simulink model "Flight_Physics2_forTrim"  (R2017b)
settings: configuration reference "cs" (kept outside this file)
undefined symbols (not defined in the file or in its folder): Configuration, FOR_LDG_R_B, g, MOM_LDG_R_B, Ts
libraries: MathLibrary x2
settings Model: Creator=zht  LastModifiedBy=One
settings ConfigSetRef: SourceLocation=Base Workspace

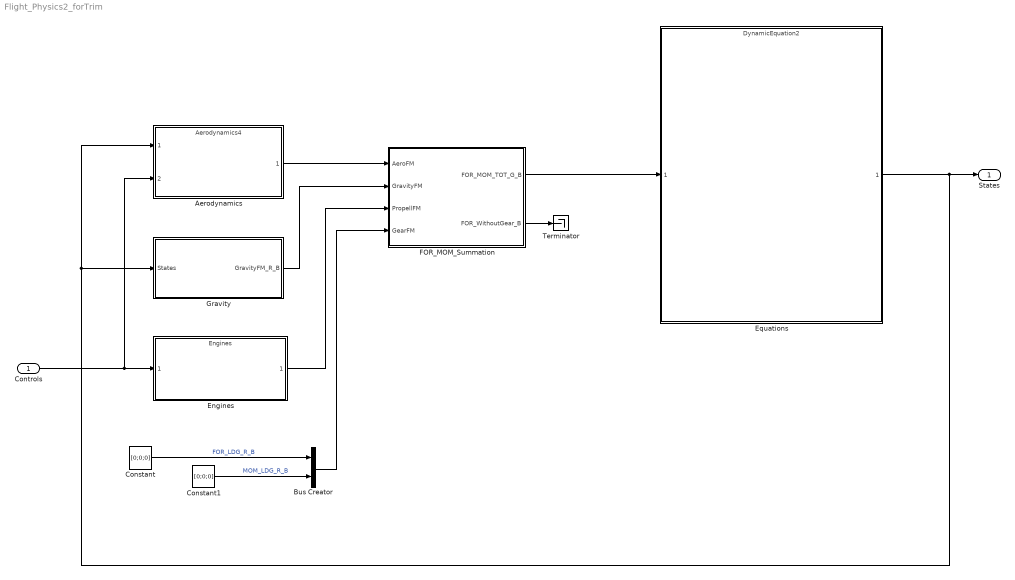
== system Flight_Physics2_forTrim ==
  Controls : Inport  OutDataTypeStr=Bus: Controls_CMD_BUS
  Aerodynamics : ModelReference  ModelNameDialog=Aerodynamics4.slx  SimulationMode=Normal  ModelReferenceVersion=1.43
  Bus Creator : BusCreator  Inputs=FOR_LDG_R_B,MOM_LDG_R_B  OutDataTypeStr=Bus: GearFM_BUS  NonVirtualBus=on
  Constant : Constant  Value=[0;0;0]
  Constant1 : Constant  Value=[0;0;0]
  Engines : ModelReference  ModelNameDialog=Engines.slx  SimulationMode=Normal  ModelReferenceVersion=1.21
  Equations : ModelReference  ModelNameDialog=DynamicEquation2  SimulationMode=Normal  ModelReferenceVersion=1.41
  FOR_MOM_Summation : Subsystem
  Gravity : Subsystem
  Terminator : Terminator
  States : Outport  OutDataTypeStr=Bus: States_BUS
  wires:
  Controls/1 -> Aerodynamics/2, Engines/1
  FOR_MOM_Summation/1(FOR_MOM_TOT_G_B) -> Equations/1
  Aerodynamics/1 -> FOR_MOM_Summation/1(AeroFM)
  Bus Creator/1 -> FOR_MOM_Summation/4(GearFM)
  Gravity/1(GravityFM_R_B) -> FOR_MOM_Summation/2(GravityFM)
  Engines/1 -> FOR_MOM_Summation/3(PropellFM)
  Constant/1 -> Bus Creator/1  "FOR_LDG_R_B"
  Constant1/1 -> Bus Creator/2  "MOM_LDG_R_B"
  FOR_MOM_Summation/2(FOR_WithoutGear_B) -> Terminator/1
  Equations/1 -> Aerodynamics/1, Gravity/1(States), States/1

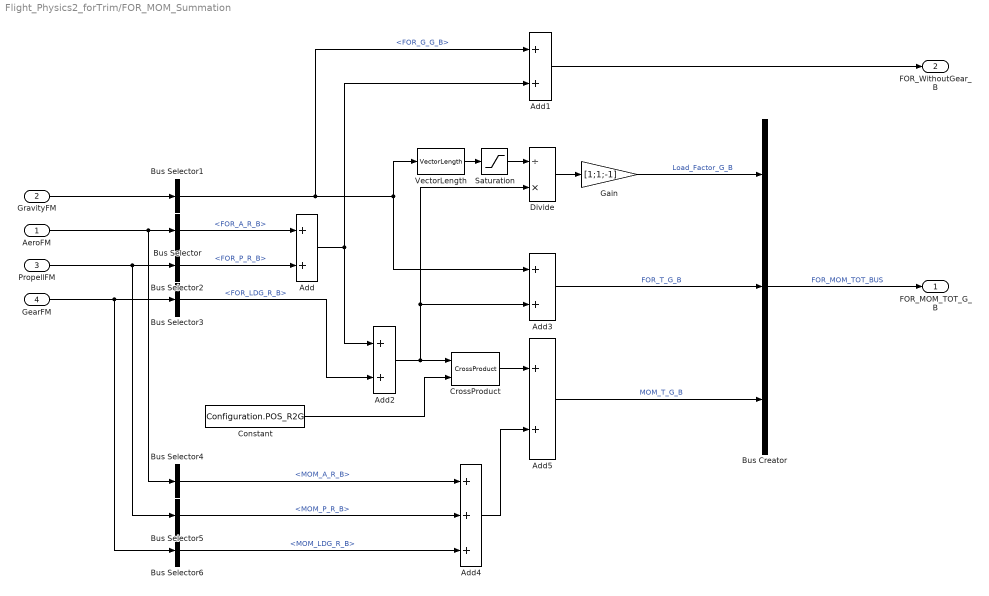
== system Flight_Physics2_forTrim/FOR_MOM_Summation ==
  AeroFM : Inport  OutDataTypeStr=Bus: AeroFM_BUS
  GravityFM : Inport  Port=2  OutDataTypeStr=Bus: GravityFM_BUS
  PropellFM : Inport  Port=3  OutDataTypeStr=Bus: PropellFM_BUS
  GearFM : Inport  Port=4  OutDataTypeStr=Bus: GearFM_BUS
  Add{,1..3,5} (5 alike) : Sum
  Add4 : Sum  Inputs=+++
  Bus Creator : BusCreator  Inputs=3  OutDataTypeStr=Bus: FOR_MOM_TOT_BUS
  Bus Selector : BusSelector  OutputSignals=FOR_A_R_B
  Bus Selector1 : BusSelector  OutputSignals=FOR_G_G_B
  Bus Selector2 : BusSelector  OutputSignals=FOR_P_R_B
  Bus Selector3 : BusSelector  OutputSignals=FOR_LDG_R_B
  Bus Selector4 : BusSelector  OutputSignals=MOM_A_R_B
  Bus Selector5 : BusSelector  OutputSignals=MOM_P_R_B
  Bus Selector6 : BusSelector  OutputSignals=MOM_LDG_R_B
  Constant : Constant  Value=Configuration.POS_R2G
  CrossProduct : MathLibrary/CrossProduct
  Divide : Product  Inputs=/*
  Gain : Gain  Gain=[1;1;-1]
  Saturation : Saturate  UpperLimit=inf  LowerLimit=0.01
  VectorLength : MathLibrary/VectorLength
  FOR_MOM_TOT_G_B : Outport  OutDataTypeStr=Bus: FOR_MOM_TOT_BUS
  FOR_WithoutGear_B : Outport  Port=2
  wires:
  PropellFM/1 -> Bus Selector5/1, Bus Selector2/1
  AeroFM/1 -> Bus Selector4/1, Bus Selector/1
  GravityFM/1 -> Bus Selector1/1
  GearFM/1 -> Bus Selector3/1, Bus Selector6/1
  Bus Creator/1 -> FOR_MOM_TOT_G_B/1  "FOR_MOM_TOT_BUS"
  Add1/1 -> FOR_WithoutGear_B/1
  Bus Selector/1 -> Add/1  "<FOR_A_R_B>"
  Bus Selector2/1 -> Add/2  "<FOR_P_R_B>"
  Add/1 -> Add2/1, Add1/2
  Bus Selector1/1 -> Add1/1, VectorLength/1, Add3/1  "<FOR_G_G_B>"
  Bus Selector3/1 -> Add2/2  "<FOR_LDG_R_B>"
  Add2/1 -> CrossProduct/1, Divide/2, Add3/2
  VectorLength/1 -> Saturation/1
  Divide/1 -> Gain/1
  Gain/1 -> Bus Creator/1  "Load_Factor_G_B"
  Add3/1 -> Bus Creator/2  "FOR_T_G_B"
  Bus Selector4/1 -> Add4/1  "<MOM_A_R_B>"
  Bus Selector5/1 -> Add4/2  "<MOM_P_R_B>"
  Bus Selector6/1 -> Add4/3  "<MOM_LDG_R_B>"
  CrossProduct/1 -> Add5/1
  Add4/1 -> Add5/2
  Add5/1 -> Bus Creator/3  "MOM_T_G_B"
  Constant/1 -> CrossProduct/2
  Saturation/1 -> Divide/1

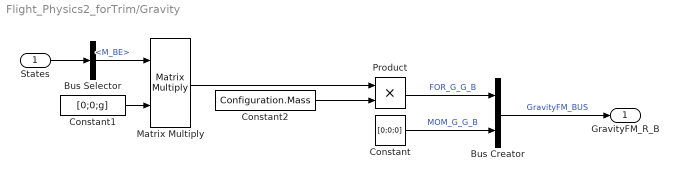
== system Flight_Physics2_forTrim/Gravity ==
  States : Inport  OutDataTypeStr=Bus: States_BUS
  Bus Creator : BusCreator  Inputs=2  OutDataTypeStr=Bus: GravityFM_BUS
  Bus Selector : BusSelector  OutputSignals=M_BE
  Constant : Constant  Value=[0;0;0]
  Constant1 : Constant  Value=[0;0;g]  SampleTime=Ts
  Constant2 : Constant  Value=Configuration.Mass  SampleTime=Ts
  Matrix Multiply : Product  Multiplication=Matrix(*)
  Product : Product
  GravityFM_R_B : Outport  OutDataTypeStr=Bus: GravityFM_BUS
  wires:
  States/1 -> Bus Selector/1
  Bus Selector/1 -> Matrix Multiply/1  "<M_BE>"
  Constant1/1 -> Matrix Multiply/2
  Matrix Multiply/1 -> Product/1
  Constant2/1 -> Product/2
  Product/1 -> Bus Creator/1  "FOR_G_G_B"
  Constant/1 -> Bus Creator/2  "MOM_G_G_B"
  Bus Creator/1 -> GravityFM_R_B/1  "GravityFM_BUS"
